simulink model "sim_tutorial2"  (Simulink 10.0)
settings: Solver=ode23tb  StartTime=0.0  StopTime=100  RelTol=1e-3  AbsTol=1e-4  EnableMultiTasking=on
undefined symbols (not defined in the file): a, b, bu, c, d, du, Rot
libraries: simulink3 x3
settings Model: Creator=bhisma  LastModifiedBy=bhisma  ExtModeTrigMode=oneshot  ExtModeArmWhenConnect=off
settings DataIOCC: SignalLoggingSaveFormat=ModelDataLogs
settings OptimizationCC: BlockReduction=off  BooleanDataType=off  LifeSpan=auto
settings DebuggingCC: SaveWithParameterizedLinksMsg=none  SignalResolutionControl=TryResolveAllWithWarning  MultiTaskDSMMsg=warning  MultiTaskCondExecSysMsg=none  SFUnexpectedBacktrackingDiag=error  SFNoUnconditionalDefaultTransitionDiag=error  SFExecutionAtInitializationDiag=warning  ArithmeticOperatorsInVariantConditions=error
settings HardwareCC: ProdBitPerPointer=64  ProdBitPerSizeT=64  ProdBitPerPtrDiffT=64  ProdLargestAtomicFloat=Float  ProdIntDivRoundTo=Zero  ProdEndianess=LittleEndian  ProdWordSize=64  ProdHWDeviceType=Intel->x86-64 (Windows64)  TargetUnknown=on
settings SFSimCC: SimUseLocalCustomCode=on  CustomCodeUndefinedFunction=FilterOut
settings RTWCC: RTWUseLocalCustomCode=on
settings CodeAppCC: StateflowObjectComments=off
settings GRTTargetCC: TargetLangStandard=C99 (ISO)
settings ConfigComp: CovMetricSettings=dwe  CovHtmlReporting=off  CovSaveCumulativeToWorkspaceVar=off  CovSaveSingleToWorkspaceVar=off

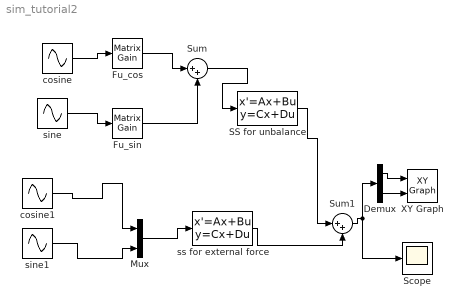
== system sim_tutorial2 ==
  Demux : Demux  Outputs=2
  Fu_cos : simulink3/Math/Matrix Gain  K=Rot.Fu_cos
      settings: SourceProductName=Simulink  SourceProductBaseCode=SL
  Fu_sin : simulink3/Math/Matrix Gain  K=Rot.Fu_sin
      settings: SourceProductName=Simulink  SourceProductBaseCode=SL
  Mux : Mux  Inputs=2
  SS for unbalance : StateSpace  A=a  B=bu  C=c  D=du  InitialCondition=0
  Scope : Scope
  Sum : Sum  Inputs=|++  SaturateOnIntegerOverflow=on  InputSameDT=on  OutDataTypeStr=Inherit: Same as first input
  Sum1 : Sum  Inputs=|++  SaturateOnIntegerOverflow=on  InputSameDT=on  OutDataTypeStr=Inherit: Same as first input
  XY Graph : simulink3/Sinks/XY Graph  xmin=-1e-2  xmax=1e-2  ymin=-1e-2  ymax=1e-2  st=-1
      settings: SourceProductName=Simulink  SourceProductBaseCode=SL
  cosine : Sin  Frequency=Rot.W  Phase=pi/2  SampleTime=0
  cosine1 : Sin  Frequency=1.21  Phase=pi/2  SampleTime=0
  sine : Sin  Frequency=Rot.W  SampleTime=0
  sine1 : Sin  SampleTime=0
  ss for external force : StateSpace  A=a  B=b  C=c  D=d  InitialCondition=0
  wires:
  cosine/1 -> Fu_cos/1
  sine/1 -> Fu_sin/1
  Sum/1 -> SS for unbalance/1
  Fu_cos/1 -> Sum/1
  Fu_sin/1 -> Sum/2
  Mux/1 -> ss for external force/1
  ss for external force/1 -> Sum1/2
  Sum1/1 -> Scope/1, Demux/1
  Demux/2 -> XY Graph/2
  Demux/1 -> XY Graph/1
  SS for unbalance/1 -> Sum1/1
  sine1/1 -> Mux/2
  cosine1/1 -> Mux/1
